simulink model "kadai34"  (R2021b)
settings: Solver=VariableStepAuto  StartTime=0.0  StopTime=5000  MaxStep=0.01  RelTol=1e-3
settings Model: Creator=tomotomo  LastModifiedBy=tomotomo

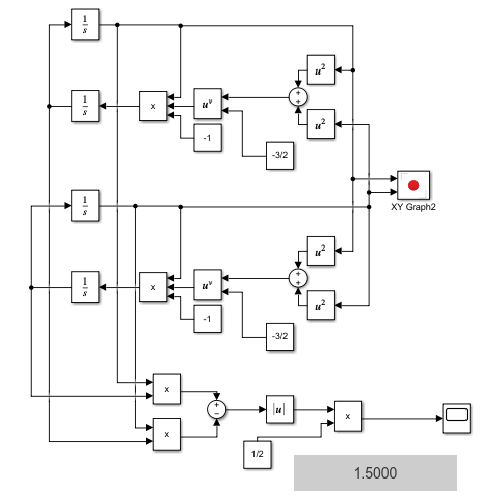
[thumbnail: Simulink's stored preview of the top-level diagram]
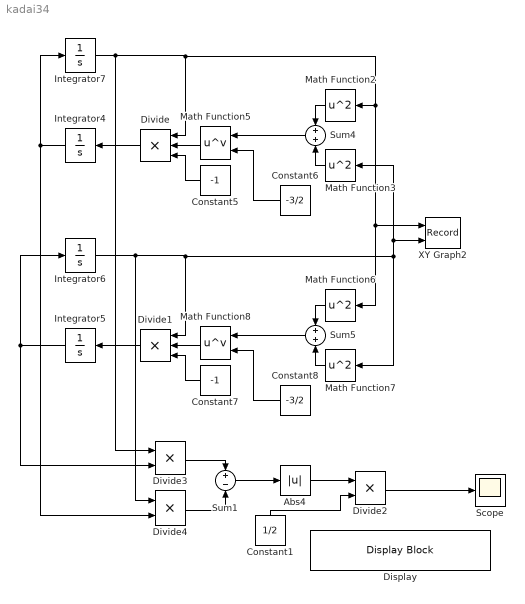
== system kadai34 ==
  Abs4 : Abs
  Constant1 : Constant  Value=1/2
  Constant5 : Constant  Value=-1
  Constant6 : Constant  Value=-3/2
  Constant7 : Constant  Value=-1
  Constant8 : Constant  Value=-3/2
  Display : DisplayBlock  LabelPosition=Hide  Format=short  Transparency=1
  Divide : Product  Inputs=***
  Divide1 : Product  Inputs=***
  Divide2 : Product  Inputs=**
  Divide3 : Product  Inputs=**
  Divide4 : Product  Inputs=**
  Integrator4 : Integrator  InitialCondition=0.15
  Integrator5 : Integrator  InitialCondition=0.0
  Integrator6 : Integrator  InitialCondition=20.0
  Integrator7 : Integrator  InitialCondition=0.0
  Math Function{2..3,6..7} (4 alike) : Math  Operator=square  SaturateOnIntegerOverflow=on
  Math Function5 : Math  Operator=pow  SaturateOnIntegerOverflow=on
  Math Function8 : Math  Operator=pow  SaturateOnIntegerOverflow=on
  Scope : Scope
  Sum1 : Sum  Inputs=+|-
  Sum4 : Sum  Inputs=+|+
  Sum5 : Sum  Inputs=+|+
  XY Graph2 : Record  FileSettingsInternal="{\"entries\":[{\"content\":{\"excelSettings\":{\"content\":{},\"type\":\"Streamout.ExcelSettings\"}},\"type\":\"Streamout.FileSettingStorage\",\"uuid\":\"9004cf79-980c-48ce-b532-17cc8f7c39f4\"}],\"packageUris\":[\"http://schema.mathworks.com/mf0/streamout_blocks/R2020a\"],\"version\":\"1.0\"}"  Layout=[1 1]  SignalsInternal="{\"entries\":[{\"content\":{\"signals\":[{\"content\":{\"blockPath\":[\"kadai34/XY Graph2\"],\"channel\":[],\"dimensions\":[1],\"domain\":\"kadai34/XY Graph2\",\"lineColor\":\"#a2142f\",\"plots\":[1],\"port\":1,\"sid\":[\"\"],\"signalID\":1166,\"signalName\":\"Integrator7\"},\"type\":\"RecordBlkView.Signal\",\"uuid\":\"e9c5ead5-75b0-4802-8505-fc29f1c6cd0d\"},{\"content\":{\"blockPath\":[\"kadai34/XY Graph2\"],\"channel\":[],\"dimensions\":[1],\"domain\":\"kadai34/XY Graph2\",\"lineColor\":\"#139fff\",\"plots\":[1],\"port\":2,\"sid\":[\"\"],\"signalID\":1170,\"signalName\":\"Integrator6\"},\"type\":\"RecordBlkView.Signal\",\"uuid\":\"6f2d3942-e53f-44c8-b247-3ae99c14b788\"}]},\"type\":\"RecordBlkView.InputSignals\",\"uuid\":\"7977afc6-9da0-4135-b7db-fb772807bc6f\"}],\"packageUris\":[\"http://schema.mathworks.com/mf0/streamout_blocks/R2020a\"],\"version\":\"1.0\"}"  VisualizationBindings="{\"xyplotplugin\":{\"info\":[{\"series\":[{\"bindingParametersList\":[{\"parameter\":\"X-Axis\",\"signalID\":1166,\"signalName\":\"Integrator7\"},{\"parameter\":\"Y-Axis\",\"signalID\":1170,\"signalName\":\"Integrator6\"}],\"seriesID\":31053}],\"subplotID\":1}]}}"  CompatibilityTag=XY
  wires:
  Constant5/1 -> Divide/3
  Constant6/1 -> Math Function5/2
  Math Function3/1 -> Sum4/2
  Constant8/1 -> Math Function8/2
  Constant7/1 -> Divide1/3
  Sum4/1 -> Math Function5/1
  Divide/1 -> Integrator4/1
  Divide1/1 -> Integrator5/1
  Sum5/1 -> Math Function8/1
  Math Function5/1 -> Divide/2
  Math Function7/1 -> Sum5/2
  Math Function2/1 -> Sum4/1
  Math Function6/1 -> Sum5/1
  Math Function8/1 -> Divide1/2
  Divide2/1 -> Scope/1
  Divide3/1 -> Sum1/1
  Divide4/1 -> Sum1/2
  Constant1/1 -> Divide2/2
  Integrator6/1 -> Divide4/1, Divide1/1, XY Graph2/2, Math Function3/1, Math Function7/1
  Integrator4/1 -> Divide4/2, Integrator7/1
  Integrator5/1 -> Divide3/2, Integrator6/1
  Integrator7/1 -> Divide3/1, Divide/1, XY Graph2/1, Math Function6/1, Math Function2/1
  Sum1/1 -> Abs4/1
  Abs4/1 -> Divide2/1
